simulink model "equivalent"  (R2018a)
settings: Solver=VariableStepAuto  StartTime=0.0  StopTime=10.0  RelTol=1e-3
undefined symbols (not defined in the file): DiscIntNeverNeededParam, sigbuilder_block
libraries: simulink x479
(part 3 of 10)

== system equivalent/cfblk303 ==
  cfblk1 : Inport
  cfblk9 : Inport  Port=2
  Action Port : ActionPort  ActionType=then
  cfblk10 : Subsystem  TreatAsAtomicUnit=on
  cfblk11 : Subsystem  TreatAsAtomicUnit=on
  cfblk12 : Delay
  cfblk13 : Delay
  cfblk3 : DiscreteZeroPole  Poles=[0 0.5]  Gain=1  SampleTime=-1
  cfblk4 : UnitDelay  SampleTime=-1
  cfblk5 : simulink/Discrete/Tapped Delay  vinit=0.0  samptime=-1  NumDelays=1  DelayOrder=Oldest  includeCurrent=off
  cfblk6 : simulink/Discrete/Transfer Fcn Lead or Lag  PoleZ=0.95  ZeroZ=0.75  ICPrevOutput=0.0  ICPrevInput=0.0  DoSatur=off
      settings: SourceProductName=Simulink  SourceProductBaseCode=SL
  cfblk7 : simulink/Discrete/Transfer Fcn Lead or Lag  PoleZ=0.95  ZeroZ=0.75  ICPrevOutput=0.0  ICPrevInput=0.0  DoSatur=off
      settings: SourceProductName=Simulink  SourceProductBaseCode=SL
  cfblk8 : If  SampleTime=1
  cyemi_{597..600,612..613,626..633} (14 alike) : DataTypeConversion  OutDataTypeStr=double
  cfblk2 : Outport
  wires:
  cfblk7/1 -> cyemi_613/1, cyemi_633/1
  cfblk1/1 -> cyemi_600/1, cyemi_630/1
  cfblk10/1(cfblk2) -> cfblk2/1
  cfblk8/1 -> cfblk10/Action
  cfblk8/2 -> cfblk11/Action
  cyemi_597/1 -> cfblk10/1(cfblk1)
  cfblk3/1 -> cyemi_597/1
  cyemi_598/1 -> cfblk10/2(cfblk12)
  cfblk12/1 -> cyemi_598/1
  cyemi_599/1 -> cfblk10/3(cfblk13)
  cfblk13/1 -> cyemi_599/1
  cyemi_600/1 -> cfblk10/4(cfblk14)
  cyemi_612/1 -> cfblk11/1(cfblk1)
  cfblk10/2(cfblk15) -> cyemi_612/1
  cyemi_613/1 -> cfblk11/2(cfblk13)
  cyemi_626/1 -> cfblk12/1
  cfblk11/1(cfblk2) -> cyemi_626/1
  cyemi_627/1 -> cfblk13/1
  cfblk11/2(cfblk14) -> cyemi_627/1
  cyemi_628/1 -> cfblk3/1
  cfblk5/1 -> cyemi_628/1
  cyemi_629/1 -> cfblk4/1
  cfblk6/1 -> cyemi_629/1
  cyemi_630/1 -> cfblk5/1
  cyemi_631/1 -> cfblk6/1
  cfblk9/1 -> cyemi_631/1
  cyemi_632/1 -> cfblk7/1
  cfblk4/1 -> cyemi_632/1
  cyemi_633/1 -> cfblk8/1

== system equivalent/cfblk304 ==
  cfblk1 : Inport
  cfblk7 : Inport  Port=2
  Action Port : ActionPort  ActionType=else
  cfblk10 : Subsystem  TreatAsAtomicUnit=on
  cfblk11 : Subsystem  TreatAsAtomicUnit=on
  cfblk12 : Delay
  cfblk13 : Delay
  cfblk3 : DiscreteTransferFcn
  cfblk4 : DiscreteFir
  cfblk5 : simulink/Continuous/PID Controller  Controller=PID  TimeDomain=Discrete-time  SampleTime=-1  IntegratorMethod=Forward Euler  FilterMethod=Forward Euler  Form=Parallel  UseFilter=on  ControllerParametersSource=internal  P=1  I=1  D=0  N=100  InitialConditionSource=internal  InitialConditionForIntegrator=0  InitialConditionForFilter=0  ExternalReset=none  LimitOutput=off  UpperSaturationLimit=inf  LowerSaturationLimit=-inf  LinearizeAsGain=off  AntiWindupMode=none  Kb=1  TrackingMode=off  Kt=1  PParamMin=[]  PParamMax=[]  IParamMin=[]  IParamMax=[]  DParamMin=[]  DParamMax=[]  NParamMin=[]  NParamMax=[]  KbParamMin=[]  KbParamMax=[]  KtParamMin=[]  KtParamMax=[]  POutMin=[]  POutMax=[]  IOutMin=[]  IOutMax=[]  DOutMin=[]  DOutMax=[]  NOutMin=[]  NOutMax=[]  KbOutMin=[]  KbOutMax=[]  KtOutMin=[]  KtOutMax=[]  IntegratorOutMin=[]  IntegratorOutMax=[]  FilterOutMin=[]  FilterOutMax=[]  SumOutMin=[]  SumOutMax=[]  SumI1OutMin=[]  SumI1OutMax=[]  SumI2OutMin=[]  SumI2OutMax=[]  SumI3OutMin=[]  SumI3OutMax=[]  SumDOutMin=[]  SumDOutMax=[]  SaturationOutMin=[]  SaturationOutMax=[]  IntegratorContinuousStateAttributes=''  IntegratorStateMustResolveToSignalObject=off  IntegratorRTWStateStorageClass=Auto  FilterContinuousStateAttributes=''  FilterStateMustResolveToSignalObject=off  FilterRTWStateStorageClass=Auto  DifferentiatorICPrevScaledInput=0  DifferentiatorOutMin=[]  DifferentiatorOutMax=[]  FilterDiffOutCoefMin=[]  FilterDiffOutCoefMax=[]  SumDenOutMin=[]  SumDenOutMax=[]  SumNumOutMin=[]  SumNumOutMax=[]  ReciprocalOutMin=[]  ReciprocalOutMax=[]  DivideOutMin=[]  DivideOutMax=[]  TunerSelectOption=Transfer Function Based (PID Tuner App)
  cfblk6 : If  SampleTime=1
  cyemi_{636..637,650,657..662} (9 alike) : DataTypeConversion  OutDataTypeStr=double
  cfblk2 : Outport
  cfblk8 : Outport  Port=2
  cfblk9 : Outport  Port=3
  wires:
  cfblk4/1 -> cfblk8/1, cyemi_637/1
  cfblk5/1 -> cfblk2/1
  cfblk11/1(cfblk2) -> cfblk9/1
  cfblk11/2(cfblk7) -> cyemi_636/1, cyemi_658/1
  cfblk6/1 -> cfblk10/Action
  cfblk6/2 -> cfblk11/Action
  cyemi_636/1 -> cfblk10/1(cfblk1)
  cyemi_637/1 -> cfblk10/2(cfblk12)
  cyemi_650/1 -> cfblk11/1(cfblk1)
  cfblk7/1 -> cyemi_650/1
  cyemi_657/1 -> cfblk12/1
  cfblk10/1(cfblk2) -> cyemi_657/1
  cyemi_658/1 -> cfblk13/1
  cyemi_659/1 -> cfblk3/1
  cfblk1/1 -> cyemi_659/1
  cyemi_660/1 -> cfblk4/1
  cfblk12/1 -> cyemi_660/1
  cyemi_661/1 -> cfblk5/1
  cfblk3/1 -> cyemi_661/1
  cyemi_662/1 -> cfblk6/1
  cfblk13/1 -> cyemi_662/1

== system equivalent/cfblk305 ==
  cfblk1 : Inport
  cfblk9 : Inport  Port=2
  cfblk10 : Inport  Port=3
  cfblk11 : Inport  Port=4
  cfblk12 : Inport  Port=5
  Action Port : ActionPort  ActionType=then
  cfblk14 : Subsystem  TreatAsAtomicUnit=on
  cfblk15 : Subsystem  TreatAsAtomicUnit=on
  cfblk16 : Delay
  cfblk3 : DiscreteFir
  cfblk4 : DiscreteStateSpace  SampleTime=-1
  cfblk5 : simulink/Discrete/Tapped Delay  vinit=0.0  samptime=-1  NumDelays=1  DelayOrder=Oldest  includeCurrent=off
  cfblk6 : simulink/Discrete/Transfer Fcn Lead or Lag  PoleZ=0.95  ZeroZ=0.75  ICPrevOutput=0.0  ICPrevInput=0.0  DoSatur=off
      settings: SourceProductName=Simulink  SourceProductBaseCode=SL
  cfblk7 : simulink/Discrete/Transfer Fcn First Order  PoleZ=0.95  ICPrevOutput=0.0  DoSatur=off
      settings: SourceProductName=Simulink
  cfblk8 : If  SampleTime=1
  cyemi_{668,678..681,698..704} (12 alike) : DataTypeConversion  OutDataTypeStr=double
  cfblk2 : Outport
  cfblk13 : Outport  Port=2
  wires:
  cfblk14/1(cfblk2) -> cfblk13/1
  cfblk15/1(cfblk2) -> cfblk2/1
  cfblk8/1 -> cfblk14/Action
  cfblk8/2 -> cfblk15/Action
  cyemi_668/1 -> cfblk14/1(cfblk1)
  cfblk7/1 -> cyemi_668/1
  cyemi_678/1 -> cfblk15/1(cfblk1)
  cfblk6/1 -> cyemi_678/1
  cyemi_679/1 -> cfblk15/2(cfblk14)
  cfblk4/1 -> cyemi_679/1
  cyemi_680/1 -> cfblk15/3(cfblk15)
  cfblk5/1 -> cyemi_680/1
  cyemi_681/1 -> cfblk15/4(cfblk16)
  cfblk9/1 -> cyemi_681/1
  cyemi_698/1 -> cfblk16/1
  cfblk15/2(cfblk17) -> cyemi_698/1
  cyemi_699/1 -> cfblk3/1
  cfblk16/1 -> cyemi_699/1
  cyemi_700/1 -> cfblk4/1
  cfblk12/1 -> cyemi_700/1
  cyemi_701/1 -> cfblk5/1
  cfblk10/1 -> cyemi_701/1
  cyemi_702/1 -> cfblk6/1
  cfblk3/1 -> cyemi_702/1
  cyemi_703/1 -> cfblk7/1
  cfblk1/1 -> cyemi_703/1
  cyemi_704/1 -> cfblk8/1
  cfblk11/1 -> cyemi_704/1

== system equivalent/cfblk306 ==
  cfblk1 : Inport
  Action Port : ActionPort  ActionType=else
  cfblk10 : DiscreteFir
  cfblk11 : DiscreteZeroPole  Poles=[0 0.5]  Gain=1  SampleTime=-1
  cfblk13 : Delay
  cfblk14 : Delay
  cfblk3 : Delay  ShowEnablePort=on
      settings: InputPortMap=u0,e6
  cfblk4 : DiscreteTransferFcn
  cfblk5 : Delay  ShowEnablePort=on
      settings: InputPortMap=u0,e6
  cfblk6 : Delay  DelayLengthSource=Input port
      settings: InputPortMap=u0,p1
  cfblk7 : Delay  DelayLengthSource=Input port
      settings: InputPortMap=u0,p1
  cfblk8 : Delay  DelayLengthSource=Input port
      settings: InputPortMap=u0,p1
  cfblk9 : simulink/Continuous/PID Controller (2DOF)  Controller=PID  TimeDomain=Discrete-time  SampleTime=-1  IntegratorMethod=Forward Euler  FilterMethod=Forward Euler  Form=Parallel  UseFilter=on  ControllerParametersSource=internal  P=1  I=1  D=0  N=100  b=1  c=1  InitialConditionSource=internal  InitialConditionForIntegrator=0  InitialConditionForFilter=0  ExternalReset=none  LimitOutput=off  UpperSaturationLimit=inf  LowerSaturationLimit=-inf  LinearizeAsGain=off  AntiWindupMode=none  Kb=1  TrackingMode=off  Kt=1  PParamMin=[]  PParamMax=[]  IParamMin=[]  IParamMax=[]  DParamMin=[]  DParamMax=[]  NParamMin=[]  NParamMax=[]  bParamMin=[]  bParamMax=[]  cParamMin=[]  cParamMax=[]  KbParamMin=[]  KbParamMax=[]  KtParamMin=[]  KtParamMax=[]  POutMin=[]  POutMax=[]  IOutMin=[]  IOutMax=[]  DOutMin=[]  DOutMax=[]  NOutMin=[]  NOutMax=[]  bOutMin=[]  bOutMax=[]  cOutMin=[]  cOutMax=[]  KbOutMin=[]  KbOutMax=[]  KtOutMin=[]  KtOutMax=[]  IntegratorOutMin=[]  IntegratorOutMax=[]  FilterOutMin=[]  FilterOutMax=[]  SumOutMin=[]  SumOutMax=[]  Sum1OutMin=[]  Sum1OutMax=[]  Sum2OutMin=[]  Sum2OutMax=[]  Sum3OutMin=[]  Sum3OutMax=[]  SumI1OutMin=[]  SumI1OutMax=[]  SumI2OutMin=[]  SumI2OutMax=[]  SumI3OutMin=[]  SumI3OutMax=[]  SumDOutMin=[]  SumDOutMax=[]  SaturationOutMin=[]  SaturationOutMax=[]  IntegratorContinuousStateAttributes=''  IntegratorStateMustResolveToSignalObject=off  IntegratorRTWStateStorageClass=Auto  FilterContinuousStateAttributes=''  FilterStateMustResolveToSignalObject=off  FilterRTWStateStorageClass=Auto  DifferentiatorICPrevScaledInput=0  DifferentiatorOutMin=[]  DifferentiatorOutMax=[]  FilterDiffOutCoefMin=[]  FilterDiffOutCoefMax=[]  SumDenOutMin=[]  SumDenOutMax=[]  SumNumOutMin=[]  SumNumOutMax=[]  ReciprocalOutMin=[]  ReciprocalOutMax=[]  DivideOutMin=[]  DivideOutMax=[]  TunerSelectOption=Transfer Function Based (PID Tuner App)
  cyemi_{706..722} (17 alike) : DataTypeConversion  OutDataTypeStr=double
  cfblk2 : Outport
  cfblk12 : Outport  Port=2
  wires:
  cfblk9/1 -> cfblk2/1, cyemi_718/1
  cfblk5/1 -> cyemi_710/1, cyemi_712/1
  cfblk3/1 -> cfblk12/1, cyemi_716/1
  cfblk4/1 -> cyemi_707/1, cyemi_719/1
  cfblk1/1 -> cyemi_713/1, cyemi_720/1
  cfblk10/1 -> cyemi_709/1, cyemi_711/1, cyemi_721/1
  cyemi_706/1 -> cfblk10/1
  cfblk11/1 -> cyemi_706/1
  cyemi_707/1 -> cfblk11/1
  cyemi_708/1 -> cfblk13/1
  cfblk7/1 -> cyemi_708/1
  cyemi_709/1 -> cfblk14/1
  cyemi_710/1 -> cfblk3/1
  cyemi_711/1 -> cfblk3/2
  cyemi_712/1 -> cfblk4/1
  cyemi_713/1 -> cfblk5/1
  cyemi_714/1 -> cfblk5/2
  cfblk14/1 -> cyemi_714/1
  cyemi_715/1 -> cfblk6/1
  cfblk13/1 -> cyemi_715/1
  cyemi_716/1 -> cfblk6/2
  cyemi_717/1 -> cfblk7/1
  cfblk6/1 -> cyemi_717/1
  cyemi_718/1 -> cfblk7/2
  cyemi_719/1 -> cfblk8/1
  cyemi_720/1 -> cfblk8/2
  cyemi_721/1 -> cfblk9/1
  cyemi_722/1 -> cfblk9/2
  cfblk8/1 -> cyemi_722/1

== system equivalent/cfblk307 ==
  cfblk1 : Inport
  cfblk12 : Inport  Port=2
  cfblk13 : Inport  Port=3
  cfblk14 : Inport  Port=4
  cfblk15 : Inport  Port=5
  cfblk16 : Inport  Port=6
  Action Port : ActionPort  ActionType=then
  cfblk10 : simulink/Discrete/Transfer Fcn Real Zero  ZeroZ=0.75  ICPrevInput=0.0  DoSatur=off
      settings: SourceProductName=Simulink  SourceProductBaseCode=SL
  cfblk11 : simulink/Discrete/Transfer Fcn Real Zero  ZeroZ=0.75  ICPrevInput=0.0  DoSatur=off
      settings: SourceProductName=Simulink  SourceProductBaseCode=SL
  cfblk{7..9,17} (4 alike) : Delay
  cfblk3 : DiscreteFilter
  cfblk4 : DiscreteFir
  cfblk5 : DiscreteIntegrator  SampleTime=-1  ICPrevOutput=DiscIntNeverNeededParam  ICPrevScaledInput=DiscIntNeverNeededParam
  cfblk6 : simulink/Discrete/Transfer Fcn First Order  PoleZ=0.95  ICPrevOutput=0.0  DoSatur=off
      settings: SourceProductName=Simulink
  cyemi_{729..738} (10 alike) : DataTypeConversion  OutDataTypeStr=double
  cfblk2 : Outport
  wires:
  cfblk15/1 -> cfblk2/1
  cyemi_729/1 -> cfblk10/1
  cfblk7/1 -> cyemi_729/1
  cyemi_730/1 -> cfblk11/1
  cfblk14/1 -> cyemi_730/1
  cyemi_731/1 -> cfblk17/1
  cfblk6/1 -> cyemi_731/1
  cyemi_732/1 -> cfblk3/1
  cfblk1/1 -> cyemi_732/1
  cyemi_733/1 -> cfblk4/1
  cfblk17/1 -> cyemi_733/1
  cyemi_734/1 -> cfblk5/1
  cfblk12/1 -> cyemi_734/1
  cyemi_735/1 -> cfblk6/1
  cfblk4/1 -> cyemi_735/1
  cyemi_736/1 -> cfblk7/1
  cfblk16/1 -> cyemi_736/1
  cyemi_737/1 -> cfblk8/1
  cfblk11/1 -> cyemi_737/1
  cyemi_738/1 -> cfblk9/1
  cfblk8/1 -> cyemi_738/1

== system equivalent/cfblk308 ==
  cfblk1 : Inport
  cfblk10 : Inport  Port=2
  Action Port : ActionPort  ActionType=else
  cfblk11 : Subsystem  TreatAsAtomicUnit=on
  cfblk12 : Subsystem  TreatAsAtomicUnit=on
  cfblk{13..16} (4 alike) : Delay
  cfblk3 : DiscreteIntegrator  SampleTime=-1  ICPrevOutput=DiscIntNeverNeededParam  ICPrevScaledInput=DiscIntNeverNeededParam
  cfblk4 : simulink/Continuous/PID Controller (2DOF)  Controller=PID  TimeDomain=Discrete-time  SampleTime=-1  IntegratorMethod=Forward Euler  FilterMethod=Forward Euler  Form=Parallel  UseFilter=on  ControllerParametersSource=internal  P=1  I=1  D=0  N=100  b=1  c=1  InitialConditionSource=internal  InitialConditionForIntegrator=0  InitialConditionForFilter=0  ExternalReset=none  LimitOutput=off  UpperSaturationLimit=inf  LowerSaturationLimit=-inf  LinearizeAsGain=off  AntiWindupMode=none  Kb=1  TrackingMode=off  Kt=1  PParamMin=[]  PParamMax=[]  IParamMin=[]  IParamMax=[]  DParamMin=[]  DParamMax=[]  NParamMin=[]  NParamMax=[]  bParamMin=[]  bParamMax=[]  cParamMin=[]  cParamMax=[]  KbParamMin=[]  KbParamMax=[]  KtParamMin=[]  KtParamMax=[]  POutMin=[]  POutMax=[]  IOutMin=[]  IOutMax=[]  DOutMin=[]  DOutMax=[]  NOutMin=[]  NOutMax=[]  bOutMin=[]  bOutMax=[]  cOutMin=[]  cOutMax=[]  KbOutMin=[]  KbOutMax=[]  KtOutMin=[]  KtOutMax=[]  IntegratorOutMin=[]  IntegratorOutMax=[]  FilterOutMin=[]  FilterOutMax=[]  SumOutMin=[]  SumOutMax=[]  Sum1OutMin=[]  Sum1OutMax=[]  Sum2OutMin=[]  Sum2OutMax=[]  Sum3OutMin=[]  Sum3OutMax=[]  SumI1OutMin=[]  SumI1OutMax=[]  SumI2OutMin=[]  SumI2OutMax=[]  SumI3OutMin=[]  SumI3OutMax=[]  SumDOutMin=[]  SumDOutMax=[]  SaturationOutMin=[]  SaturationOutMax=[]  IntegratorContinuousStateAttributes=''  IntegratorStateMustResolveToSignalObject=off  IntegratorRTWStateStorageClass=Auto  FilterContinuousStateAttributes=''  FilterStateMustResolveToSignalObject=off  FilterRTWStateStorageClass=Auto  DifferentiatorICPrevScaledInput=0  DifferentiatorOutMin=[]  DifferentiatorOutMax=[]  FilterDiffOutCoefMin=[]  FilterDiffOutCoefMax=[]  SumDenOutMin=[]  SumDenOutMax=[]  SumNumOutMin=[]  SumNumOutMax=[]  ReciprocalOutMin=[]  ReciprocalOutMax=[]  DivideOutMin=[]  DivideOutMax=[]  TunerSelectOption=Transfer Function Based (PID Tuner App)
  cfblk5 : DiscreteZeroPole  Poles=[0 0.5]  Gain=1  SampleTime=-1
  cfblk6 : DiscreteFilter
  cfblk7 : DiscreteStateSpace  SampleTime=-1
  cfblk8 : simulink/Continuous/PID Controller  Controller=PID  TimeDomain=Discrete-time  SampleTime=-1  IntegratorMethod=Forward Euler  FilterMethod=Forward Euler  Form=Parallel  UseFilter=on  ControllerParametersSource=internal  P=1  I=1  D=0  N=100  InitialConditionSource=internal  InitialConditionForIntegrator=0  InitialConditionForFilter=0  ExternalReset=none  LimitOutput=off  UpperSaturationLimit=inf  LowerSaturationLimit=-inf  LinearizeAsGain=off  AntiWindupMode=none  Kb=1  TrackingMode=off  Kt=1  PParamMin=[]  PParamMax=[]  IParamMin=[]  IParamMax=[]  DParamMin=[]  DParamMax=[]  NParamMin=[]  NParamMax=[]  KbParamMin=[]  KbParamMax=[]  KtParamMin=[]  KtParamMax=[]  POutMin=[]  POutMax=[]  IOutMin=[]  IOutMax=[]  DOutMin=[]  DOutMax=[]  NOutMin=[]  NOutMax=[]  KbOutMin=[]  KbOutMax=[]  KtOutMin=[]  KtOutMax=[]  IntegratorOutMin=[]  IntegratorOutMax=[]  FilterOutMin=[]  FilterOutMax=[]  SumOutMin=[]  SumOutMax=[]  SumI1OutMin=[]  SumI1OutMax=[]  SumI2OutMin=[]  SumI2OutMax=[]  SumI3OutMin=[]  SumI3OutMax=[]  SumDOutMin=[]  SumDOutMax=[]  SaturationOutMin=[]  SaturationOutMax=[]  IntegratorContinuousStateAttributes=''  IntegratorStateMustResolveToSignalObject=off  IntegratorRTWStateStorageClass=Auto  FilterContinuousStateAttributes=''  FilterStateMustResolveToSignalObject=off  FilterRTWStateStorageClass=Auto  DifferentiatorICPrevScaledInput=0  DifferentiatorOutMin=[]  DifferentiatorOutMax=[]  FilterDiffOutCoefMin=[]  FilterDiffOutCoefMax=[]  SumDenOutMin=[]  SumDenOutMax=[]  SumNumOutMin=[]  SumNumOutMax=[]  ReciprocalOutMin=[]  ReciprocalOutMax=[]  DivideOutMin=[]  DivideOutMax=[]  TunerSelectOption=Transfer Function Based (PID Tuner App)
  cfblk9 : If  SampleTime=1
  cyemi_{741..742,750,761..772} (15 alike) : DataTypeConversion  OutDataTypeStr=double
  cfblk2 : Outport
  wires:
  cfblk1/1 -> cfblk2/1
  cfblk9/1 -> cfblk11/Action
  cfblk9/2 -> cfblk12/Action
  cyemi_741/1 -> cfblk11/1(cfblk1)
  cfblk13/1 -> cyemi_741/1
  cyemi_742/1 -> cfblk11/2(cfblk7)
  cfblk12/2(cfblk10) -> cyemi_742/1
  cyemi_750/1 -> cfblk12/1(cfblk1)
  cfblk3/1 -> cyemi_750/1
  cyemi_761/1 -> cfblk13/1
  cfblk4/1 -> cyemi_761/1
  cyemi_762/1 -> cfblk14/1
  cfblk11/1(cfblk2) -> cyemi_762/1
  cyemi_763/1 -> cfblk15/1
  cfblk7/1 -> cyemi_763/1
  cyemi_764/1 -> cfblk16/1
  cfblk6/1 -> cyemi_764/1
  cyemi_765/1 -> cfblk3/1
  cfblk8/1 -> cyemi_765/1
  cyemi_766/1 -> cfblk4/1
  cfblk12/1(cfblk2) -> cyemi_766/1
  cyemi_767/1 -> cfblk4/2
  cfblk14/1 -> cyemi_767/1
  cyemi_768/1 -> cfblk5/1
  cfblk16/1 -> cyemi_768/1
  cyemi_769/1 -> cfblk6/1
  cfblk5/1 -> cyemi_769/1
  cyemi_770/1 -> cfblk7/1
  cfblk12/3(cfblk11) -> cyemi_770/1
  cyemi_771/1 -> cfblk8/1
  cfblk10/1 -> cyemi_771/1
  cyemi_772/1 -> cfblk9/1
  cfblk15/1 -> cyemi_772/1

== system equivalent/cfblk309 ==
  cfblk1 : Inport
  cfblk13 : Inport  Port=2
  Action Port : ActionPort  ActionType=then
  cfblk10 : simulink/Continuous/PID Controller (2DOF)  Controller=PID  TimeDomain=Discrete-time  SampleTime=-1  IntegratorMethod=Forward Euler  FilterMethod=Forward Euler  Form=Parallel  UseFilter=on  ControllerParametersSource=internal  P=1  I=1  D=0  N=100  b=1  c=1  InitialConditionSource=internal  InitialConditionForIntegrator=0  InitialConditionForFilter=0  ExternalReset=none  LimitOutput=off  UpperSaturationLimit=inf  LowerSaturationLimit=-inf  LinearizeAsGain=off  AntiWindupMode=none  Kb=1  TrackingMode=off  Kt=1  PParamMin=[]  PParamMax=[]  IParamMin=[]  IParamMax=[]  DParamMin=[]  DParamMax=[]  NParamMin=[]  NParamMax=[]  bParamMin=[]  bParamMax=[]  cParamMin=[]  cParamMax=[]  KbParamMin=[]  KbParamMax=[]  KtParamMin=[]  KtParamMax=[]  POutMin=[]  POutMax=[]  IOutMin=[]  IOutMax=[]  DOutMin=[]  DOutMax=[]  NOutMin=[]  NOutMax=[]  bOutMin=[]  bOutMax=[]  cOutMin=[]  cOutMax=[]  KbOutMin=[]  KbOutMax=[]  KtOutMin=[]  KtOutMax=[]  IntegratorOutMin=[]  IntegratorOutMax=[]  FilterOutMin=[]  FilterOutMax=[]  SumOutMin=[]  SumOutMax=[]  Sum1OutMin=[]  Sum1OutMax=[]  Sum2OutMin=[]  Sum2OutMax=[]  Sum3OutMin=[]  Sum3OutMax=[]  SumI1OutMin=[]  SumI1OutMax=[]  SumI2OutMin=[]  SumI2OutMax=[]  SumI3OutMin=[]  SumI3OutMax=[]  SumDOutMin=[]  SumDOutMax=[]  SaturationOutMin=[]  SaturationOutMax=[]  IntegratorContinuousStateAttributes=''  IntegratorStateMustResolveToSignalObject=off  IntegratorRTWStateStorageClass=Auto  FilterContinuousStateAttributes=''  FilterStateMustResolveToSignalObject=off  FilterRTWStateStorageClass=Auto  DifferentiatorICPrevScaledInput=0  DifferentiatorOutMin=[]  DifferentiatorOutMax=[]  FilterDiffOutCoefMin=[]  FilterDiffOutCoefMax=[]  SumDenOutMin=[]  SumDenOutMax=[]  SumNumOutMin=[]  SumNumOutMax=[]  ReciprocalOutMin=[]  ReciprocalOutMax=[]  DivideOutMin=[]  DivideOutMax=[]  TunerSelectOption=Transfer Function Based (PID Tuner App)
  cfblk11 : DiscreteFilter
  cfblk12 : Delay
  cfblk15 : Delay
  cfblk3 : Delay  DelayLengthSource=Input port
      settings: InputPortMap=u0,p1
  cfblk4 : UnitDelay  SampleTime=-1
  cfblk5 : DiscreteStateSpace  SampleTime=-1
  cfblk6 : DiscreteZeroPole  Poles=[0 0.5]  Gain=1  SampleTime=-1
  cfblk7 : Delay  ShowEnablePort=on
      settings: InputPortMap=u0,e6
  cfblk8 : simulink/Discrete/Difference  ICPrevInput=0.0  OutMin=[]  OutMax=[]  OutDataTypeStr=Inherit: Inherit via back propagation  OutDataType=fixdt(1, 16)  OutScaling=2^-10  DoSatur=off
  cfblk9 : DiscreteTransferFcn
  cyemi_{775..788} (14 alike) : DataTypeConversion  OutDataTypeStr=double
  cfblk2 : Outport
  cfblk14 : Outport  Port=2
  wires:
  cfblk9/1 -> cyemi_785/1, cyemi_787/1
  cfblk3/1 -> cyemi_777/1, cyemi_778/1
  cfblk4/1 -> cfblk14/1
  cfblk5/1 -> cfblk2/1
  cfblk11/1 -> cyemi_786/1, cyemi_788/1
  cyemi_775/1 -> cfblk10/1
  cfblk13/1 -> cyemi_775/1
  cyemi_776/1 -> cfblk10/2
  cfblk6/1 -> cyemi_776/1
  cyemi_777/1 -> cfblk11/1
  cyemi_778/1 -> cfblk12/1
  cyemi_779/1 -> cfblk15/1
  cfblk10/1 -> cyemi_779/1
  cyemi_780/1 -> cfblk3/1
  cfblk15/1 -> cyemi_780/1
  cyemi_781/1 -> cfblk3/2
  cfblk1/1 -> cyemi_781/1
  cyemi_782/1 -> cfblk4/1
  cfblk7/1 -> cyemi_782/1
  cyemi_783/1 -> cfblk5/1
  cfblk8/1 -> cyemi_783/1
  cyemi_784/1 -> cfblk6/1
  cfblk12/1 -> cyemi_784/1
  cyemi_785/1 -> cfblk7/1
  cyemi_786/1 -> cfblk7/2
  cyemi_787/1 -> cfblk8/1
  cyemi_788/1 -> cfblk9/1

== system equivalent/cfblk310 ==
  cfblk1 : Inport
  cfblk13 : Inport  Port=2
  Action Port : ActionPort  ActionType=else
  cfblk10 : UnitDelay  SampleTime=-1
  cfblk11 : UnitDelay  SampleTime=-1
  cfblk12 : simulink/Discrete/Tapped Delay  vinit=0.0  samptime=-1  NumDelays=1  DelayOrder=Oldest  includeCurrent=off
  cfblk17 : Delay
  cfblk18 : Delay
  cfblk3 : Delay  DelayLengthSource=Input port
      settings: InputPortMap=u0,p1
  cfblk4 : DiscreteFilter
  cfblk5 : Delay
  cfblk6 : DiscreteTransferFcn
  cfblk7 : DiscreteStateSpace  SampleTime=-1
  cfblk8 : simulink/Discrete/Tapped Delay  vinit=0.0  samptime=-1  NumDelays=1  DelayOrder=Oldest  includeCurrent=off
  cfblk9 : simulink/Discrete/Tapped Delay  vinit=0.0  samptime=-1  NumDelays=1  DelayOrder=Oldest  includeCurrent=off
  cyemi_{792..804} (13 alike) : DataTypeConversion  OutDataTypeStr=double
  cfblk2 : Outport
  cfblk14 : Outport  Port=2
  cfblk15 : Outport  Port=3
  cfblk16 : Outport  Port=4
  wires:
  cfblk8/1 -> cfblk15/1
  cfblk5/1 -> cyemi_803/1, cyemi_804/1
  cfblk11/1 -> cyemi_795/1, cyemi_796/1, cyemi_802/1
  cfblk1/1 -> cfblk2/1
  cfblk7/1 -> cfblk16/1
  cfblk12/1 -> cfblk14/1
  cyemi_792/1 -> cfblk10/1
  cfblk3/1 -> cyemi_792/1
  cyemi_793/1 -> cfblk11/1
  cfblk10/1 -> cyemi_793/1
  cyemi_794/1 -> cfblk12/1
  cfblk4/1 -> cyemi_794/1
  cyemi_795/1 -> cfblk17/1
  cyemi_796/1 -> cfblk18/1
  cyemi_797/1 -> cfblk3/1
  cfblk17/1 -> cyemi_797/1
  cyemi_798/1 -> cfblk3/2
  cfblk18/1 -> cyemi_798/1
  cyemi_799/1 -> cfblk4/1
  cfblk9/1 -> cyemi_799/1
  cyemi_800/1 -> cfblk5/1
  cfblk6/1 -> cyemi_800/1
  cyemi_801/1 -> cfblk6/1
  cfblk13/1 -> cyemi_801/1
  cyemi_802/1 -> cfblk7/1
  cyemi_803/1 -> cfblk8/1
  cyemi_804/1 -> cfblk9/1

== system equivalent/cfblk311 ==
  cfblk1 : Inport
  cfblk9 : Inport  Port=2
  cfblk10 : Inport  Port=3
  cfblk11 : Inport  Port=4
  Action Port : ActionPort  ActionType=then
  cfblk3 : DiscreteFilter
  cfblk4 : DiscreteFir
  cfblk5 : simulink/Continuous/PID Controller (2DOF)  Controller=PID  TimeDomain=Discrete-time  SampleTime=-1  IntegratorMethod=Forward Euler  FilterMethod=Forward Euler  Form=Parallel  UseFilter=on  ControllerParametersSource=internal  P=1  I=1  D=0  N=100  b=1  c=1  InitialConditionSource=internal  InitialConditionForIntegrator=0  InitialConditionForFilter=0  ExternalReset=none  LimitOutput=off  UpperSaturationLimit=inf  LowerSaturationLimit=-inf  LinearizeAsGain=off  AntiWindupMode=none  Kb=1  TrackingMode=off  Kt=1  PParamMin=[]  PParamMax=[]  IParamMin=[]  IParamMax=[]  DParamMin=[]  DParamMax=[]  NParamMin=[]  NParamMax=[]  bParamMin=[]  bParamMax=[]  cParamMin=[]  cParamMax=[]  KbParamMin=[]  KbParamMax=[]  KtParamMin=[]  KtParamMax=[]  POutMin=[]  POutMax=[]  IOutMin=[]  IOutMax=[]  DOutMin=[]  DOutMax=[]  NOutMin=[]  NOutMax=[]  bOutMin=[]  bOutMax=[]  cOutMin=[]  cOutMax=[]  KbOutMin=[]  KbOutMax=[]  KtOutMin=[]  KtOutMax=[]  IntegratorOutMin=[]  IntegratorOutMax=[]  FilterOutMin=[]  FilterOutMax=[]  SumOutMin=[]  SumOutMax=[]  Sum1OutMin=[]  Sum1OutMax=[]  Sum2OutMin=[]  Sum2OutMax=[]  Sum3OutMin=[]  Sum3OutMax=[]  SumI1OutMin=[]  SumI1OutMax=[]  SumI2OutMin=[]  SumI2OutMax=[]  SumI3OutMin=[]  SumI3OutMax=[]  SumDOutMin=[]  SumDOutMax=[]  SaturationOutMin=[]  SaturationOutMax=[]  IntegratorContinuousStateAttributes=''  IntegratorStateMustResolveToSignalObject=off  IntegratorRTWStateStorageClass=Auto  FilterContinuousStateAttributes=''  FilterStateMustResolveToSignalObject=off  FilterRTWStateStorageClass=Auto  DifferentiatorICPrevScaledInput=0  DifferentiatorOutMin=[]  DifferentiatorOutMax=[]  FilterDiffOutCoefMin=[]  FilterDiffOutCoefMax=[]  SumDenOutMin=[]  SumDenOutMax=[]  SumNumOutMin=[]  SumNumOutMax=[]  ReciprocalOutMin=[]  ReciprocalOutMax=[]  DivideOutMin=[]  DivideOutMax=[]  TunerSelectOption=Transfer Function Based (PID Tuner App)
  cfblk6 : simulink/Discrete/Transfer Fcn Lead or Lag  PoleZ=0.95  ZeroZ=0.75  ICPrevOutput=0.0  ICPrevInput=0.0  DoSatur=off
      settings: SourceProductName=Simulink  SourceProductBaseCode=SL
  cfblk7 : UnitDelay  SampleTime=-1
  cfblk8 : DiscreteIntegrator  SampleTime=-1  ICPrevOutput=DiscIntNeverNeededParam  ICPrevScaledInput=DiscIntNeverNeededParam
  cyemi_{809..815} (7 alike) : DataTypeConversion  OutDataTypeStr=double
  cfblk2 : Outport
  cfblk12 : Outport  Port=2
  cfblk13 : Outport  Port=3
  wires:
  cfblk11/1 -> cfblk12/1
  cfblk4/1 -> cfblk2/1
  cfblk3/1 -> cfblk13/1
  cyemi_809/1 -> cfblk3/1
  cfblk1/1 -> cyemi_809/1
  cyemi_810/1 -> cfblk4/1
  cfblk6/1 -> cyemi_810/1
  cyemi_811/1 -> cfblk5/1
  cfblk9/1 -> cyemi_811/1
  cyemi_812/1 -> cfblk5/2
  cfblk7/1 -> cyemi_812/1
  cyemi_813/1 -> cfblk6/1
  cfblk5/1 -> cyemi_813/1
  cyemi_814/1 -> cfblk7/1
  cfblk8/1 -> cyemi_814/1
  cyemi_815/1 -> cfblk8/1
  cfblk10/1 -> cyemi_815/1

== system equivalent/cfblk312 ==
  cfblk1 : Inport
  cfblk10 : Inport  Port=2
  Action Port : ActionPort  ActionType=else
  cfblk11 : Delay
  cfblk3 : Delay  ShowEnablePort=on
      settings: InputPortMap=u0,e6
  cfblk4 : simulink/Discrete/Transfer Fcn Lead or Lag  PoleZ=0.95  ZeroZ=0.75  ICPrevOutput=0.0  ICPrevInput=0.0  DoSatur=off
      settings: SourceProductName=Simulink  SourceProductBaseCode=SL
  cfblk5 : UnitDelay  SampleTime=-1
  cfblk6 : simulink/Discrete/Transfer Fcn Real Zero  ZeroZ=0.75  ICPrevInput=0.0  DoSatur=off
      settings: SourceProductName=Simulink  SourceProductBaseCode=SL
  cfblk7 : DiscreteStateSpace  SampleTime=-1
  cfblk8 : simulink/Discrete/Transfer Fcn Lead or Lag  PoleZ=0.95  ZeroZ=0.75  ICPrevOutput=0.0  ICPrevInput=0.0  DoSatur=off
      settings: SourceProductName=Simulink  SourceProductBaseCode=SL
  cfblk9 : UnitDelay  SampleTime=-1
  cyemi_{818..826} (9 alike) : DataTypeConversion  OutDataTypeStr=double
  cfblk2 : Outport
  wires:
  cfblk4/1 -> cfblk2/1
  cyemi_818/1 -> cfblk11/1
  cfblk7/1 -> cyemi_818/1
  cyemi_819/1 -> cfblk3/1
  cfblk10/1 -> cyemi_819/1
  cyemi_820/1 -> cfblk3/2
  cfblk11/1 -> cyemi_820/1
  cyemi_821/1 -> cfblk4/1
  cfblk8/1 -> cyemi_821/1
  cyemi_822/1 -> cfblk5/1
  cfblk3/1 -> cyemi_822/1
  cyemi_823/1 -> cfblk6/1
  cfblk5/1 -> cyemi_823/1
  cyemi_824/1 -> cfblk7/1
  cfblk6/1 -> cyemi_824/1
  cyemi_825/1 -> cfblk8/1
  cfblk9/1 -> cyemi_825/1
  cyemi_826/1 -> cfblk9/1
  cfblk1/1 -> cyemi_826/1

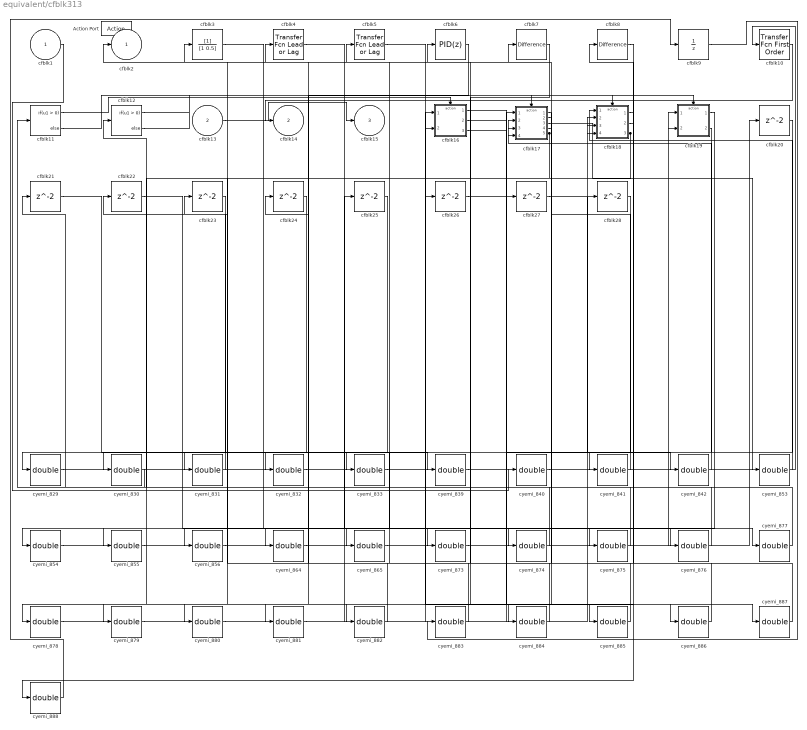
== system equivalent/cfblk313 ==
  cfblk1 : Inport
  cfblk13 : Inport  Port=2
  Action Port : ActionPort  ActionType=then
  cfblk10 : simulink/Discrete/Transfer Fcn First Order  PoleZ=0.95  ICPrevOutput=0.0  DoSatur=off
      settings: SourceProductName=Simulink
  cfblk11 : If  SampleTime=1
  cfblk12 : If  SampleTime=1
  cfblk16 : Subsystem  TreatAsAtomicUnit=on
  cfblk17 : Subsystem  TreatAsAtomicUnit=on
  cfblk18 : Subsystem  TreatAsAtomicUnit=on
  cfblk19 : Subsystem  TreatAsAtomicUnit=on
  cfblk{20..28} (9 alike) : Delay
  cfblk3 : DiscreteFilter
  cfblk4 : simulink/Discrete/Transfer Fcn Lead or Lag  PoleZ=0.95  ZeroZ=0.75  ICPrevOutput=0.0  ICPrevInput=0.0  DoSatur=off
      settings: SourceProductName=Simulink  SourceProductBaseCode=SL
  cfblk5 : simulink/Discrete/Transfer Fcn Lead or Lag  PoleZ=0.95  ZeroZ=0.75  ICPrevOutput=0.0  ICPrevInput=0.0  DoSatur=off
      settings: SourceProductName=Simulink  SourceProductBaseCode=SL
  cfblk6 : simulink/Continuous/PID Controller  Controller=PID  TimeDomain=Discrete-time  SampleTime=-1  IntegratorMethod=Forward Euler  FilterMethod=Forward Euler  Form=Parallel  UseFilter=on  ControllerParametersSource=internal  P=1  I=1  D=0  N=100  InitialConditionSource=internal  InitialConditionForIntegrator=0  InitialConditionForFilter=0  ExternalReset=none  LimitOutput=off  UpperSaturationLimit=inf  LowerSaturationLimit=-inf  LinearizeAsGain=off  AntiWindupMode=none  Kb=1  TrackingMode=off  Kt=1  PParamMin=[]  PParamMax=[]  IParamMin=[]  IParamMax=[]  DParamMin=[]  DParamMax=[]  NParamMin=[]  NParamMax=[]  KbParamMin=[]  KbParamMax=[]  KtParamMin=[]  KtParamMax=[]  POutMin=[]  POutMax=[]  IOutMin=[]  IOutMax=[]  DOutMin=[]  DOutMax=[]  NOutMin=[]  NOutMax=[]  KbOutMin=[]  KbOutMax=[]  KtOutMin=[]  KtOutMax=[]  IntegratorOutMin=[]  IntegratorOutMax=[]  FilterOutMin=[]  FilterOutMax=[]  SumOutMin=[]  SumOutMax=[]  SumI1OutMin=[]  SumI1OutMax=[]  SumI2OutMin=[]  SumI2OutMax=[]  SumI3OutMin=[]  SumI3OutMax=[]  SumDOutMin=[]  SumDOutMax=[]  SaturationOutMin=[]  SaturationOutMax=[]  IntegratorContinuousStateAttributes=''  IntegratorStateMustResolveToSignalObject=off  IntegratorRTWStateStorageClass=Auto  FilterContinuousStateAttributes=''  FilterStateMustResolveToSignalObject=off  FilterRTWStateStorageClass=Auto  DifferentiatorICPrevScaledInput=0  DifferentiatorOutMin=[]  DifferentiatorOutMax=[]  FilterDiffOutCoefMin=[]  FilterDiffOutCoefMax=[]  SumDenOutMin=[]  SumDenOutMax=[]  SumNumOutMin=[]  SumNumOutMax=[]  ReciprocalOutMin=[]  ReciprocalOutMax=[]  DivideOutMin=[]  DivideOutMax=[]  TunerSelectOption=Transfer Function Based (PID Tuner App)
  cfblk7 : simulink/Discrete/Difference  ICPrevInput=0.0  OutMin=[]  OutMax=[]  OutDataTypeStr=Inherit: Inherit via back propagation  OutDataType=fixdt(1, 16)  OutScaling=2^-10  DoSatur=off
  cfblk8 : simulink/Discrete/Difference  ICPrevInput=0.0  OutMin=[]  OutMax=[]  OutDataTypeStr=Inherit: Inherit via back propagation  OutDataType=fixdt(1, 16)  OutScaling=2^-10  DoSatur=off
  cfblk9 : UnitDelay  SampleTime=-1
  cyemi_{829..833,839..842,853..856,864..865,873..888} (31 alike) : DataTypeConversion  OutDataTypeStr=double
  cfblk2 : Outport
  cfblk14 : Outport  Port=2
  cfblk15 : Outport  Port=3
  wires:
  cfblk13/1 -> cfblk15/1
  cfblk17/2(cfblk13) -> cfblk2/1
  cfblk10/1 -> cfblk14/1
  cfblk17/5(cfblk16) -> cyemi_832/1, cyemi_856/1
  cfblk18/3(cfblk12) -> cyemi_879/1, cyemi_880/1
  cfblk11/1 -> cfblk16/Action
  cfblk11/2 -> cfblk17/Action
  cfblk12/1 -> cfblk18/Action
  cfblk12/2 -> cfblk19/Action
  cyemi_829/1 -> cfblk10/1
  cfblk19/2(cfblk10) -> cyemi_829/1
  cyemi_830/1 -> cfblk11/1
  cfblk24/1 -> cyemi_830/1
  cyemi_831/1 -> cfblk12/1
  cfblk17/1(cfblk2) -> cyemi_831/1
  cyemi_832/1 -> cfblk16/1(cfblk1)
  cyemi_833/1 -> cfblk16/2(cfblk7)
  cfblk25/1 -> cyemi_833/1
  cyemi_839/1 -> cfblk17/1(cfblk1)
  cfblk21/1 -> cyemi_839/1
  cyemi_840/1 -> cfblk17/2(cfblk10)
  cfblk1/1 -> cyemi_840/1
  cyemi_841/1 -> cfblk17/3(cfblk11)
  cfblk26/1 -> cyemi_841/1
  cyemi_842/1 -> cfblk17/4(cfblk12)
  cfblk27/1 -> cyemi_842/1
  cyemi_853/1 -> cfblk18/1(cfblk1)
  cfblk17/3(cfblk14) -> cyemi_853/1
  cyemi_854/1 -> cfblk18/2(cfblk8)
  cfblk17/4(cfblk15) -> cyemi_854/1
  cyemi_855/1 -> cfblk18/3(cfblk9)
  cfblk23/1 -> cyemi_855/1
  cyemi_856/1 -> cfblk18/4(cfblk10)
  cyemi_864/1 -> cfblk19/1(cfblk1)
  cfblk22/1 -> cyemi_864/1
  cyemi_865/1 -> cfblk19/2(cfblk9)
  cfblk20/1 -> cyemi_865/1
  cyemi_873/1 -> cfblk20/1
  cfblk3/1 -> cyemi_873/1
  cyemi_874/1 -> cfblk21/1
  cfblk19/1(cfblk2) -> cyemi_874/1
  cyemi_875/1 -> cfblk22/1
  cfblk16/2(cfblk8) -> cyemi_875/1
  cyemi_876/1 -> cfblk23/1
  cfblk16/3(cfblk9) -> cyemi_876/1
  cyemi_877/1 -> cfblk24/1
  cfblk4/1 -> cyemi_877/1
  cyemi_878/1 -> cfblk25/1
  cfblk18/2(cfblk11) -> cyemi_878/1
  cyemi_879/1 -> cfblk26/1
  cyemi_880/1 -> cfblk27/1
  cyemi_881/1 -> cfblk28/1
  cfblk6/1 -> cyemi_881/1
  cyemi_882/1 -> cfblk3/1
  cfblk7/1 -> cyemi_882/1
  cyemi_883/1 -> cfblk4/1
  cfblk9/1 -> cyemi_883/1
  cyemi_884/1 -> cfblk5/1
  cfblk28/1 -> cyemi_884/1
  cyemi_885/1 -> cfblk6/1
  cfblk8/1 -> cyemi_885/1
  cyemi_886/1 -> cfblk7/1
  cfblk16/1(cfblk2) -> cyemi_886/1
  cyemi_887/1 -> cfblk8/1
  cfblk5/1 -> cyemi_887/1
  cyemi_888/1 -> cfblk9/1
  cfblk18/1(cfblk2) -> cyemi_888/1

== system equivalent/cfblk314 ==
  cfblk1 : Inport
  Action Port : ActionPort  ActionType=else
  cfblk10 : Subsystem  TreatAsAtomicUnit=on
  cfblk11 : Subsystem  TreatAsAtomicUnit=on
  cfblk{12..15} (4 alike) : Delay
  cfblk3 : Delay  DelayLengthSource=Input port
      settings: InputPortMap=u0,p1
  cfblk4 : simulink/Discrete/Difference  ICPrevInput=0.0  OutMin=[]  OutMax=[]  OutDataTypeStr=Inherit: Inherit via back propagation  OutDataType=fixdt(1, 16)  OutScaling=2^-10  DoSatur=off
  cfblk5 : DiscreteFilter
  cfblk6 : Delay  ShowEnablePort=on
      settings: InputPortMap=u0,e6
  cfblk7 : If  SampleTime=1
  cyemi_{890..891,897..898,918..928} (15 alike) : DataTypeConversion  OutDataTypeStr=double
  cfblk2 : Outport
  cfblk8 : Outport  Port=2
  cfblk9 : Outport  Port=3
  wires:
  cfblk3/1 -> cfblk8/1, cyemi_890/1
  cfblk10/1(cfblk2) -> cfblk2/1, cyemi_897/1
  cfblk5/1 -> cfblk9/1, cyemi_921/1
  cfblk11/1(cfblk2) -> cyemi_919/1, cyemi_920/1, cyemi_925/1
  cfblk4/1 -> cyemi_918/1, cyemi_922/1, cyemi_928/1
  cfblk7/1 -> cfblk10/Action
  cfblk7/2 -> cfblk11/Action
  cyemi_890/1 -> cfblk10/1(cfblk1)
  cyemi_891/1 -> cfblk10/2(cfblk7)
  cfblk13/1 -> cyemi_891/1
  cyemi_897/1 -> cfblk11/1(cfblk1)
  cyemi_898/1 -> cfblk11/2(cfblk17)
  cfblk15/1 -> cyemi_898/1
  cyemi_918/1 -> cfblk12/1
  cyemi_919/1 -> cfblk13/1
  cyemi_920/1 -> cfblk14/1
  cyemi_921/1 -> cfblk15/1
  cyemi_922/1 -> cfblk3/1
  cyemi_923/1 -> cfblk3/2
  cfblk14/1 -> cyemi_923/1
  cyemi_924/1 -> cfblk4/1
  cfblk6/1 -> cyemi_924/1
  cyemi_925/1 -> cfblk5/1
  cyemi_926/1 -> cfblk6/1
  cfblk12/1 -> cyemi_926/1
  cyemi_927/1 -> cfblk6/2
  cfblk1/1 -> cyemi_927/1
  cyemi_928/1 -> cfblk7/1

== system equivalent/cfblk315 ==
  cfblk1 : Inport
  cfblk8 : Inport  Port=2
  cfblk9 : Inport  Port=3
  cfblk10 : Inport  Port=4
  Action Port : ActionPort  ActionType=then
  cfblk14 : Subsystem  TreatAsAtomicUnit=on
  cfblk15 : Subsystem  TreatAsAtomicUnit=on
  cfblk3 : simulink/Discrete/Transfer Fcn Real Zero  ZeroZ=0.75  ICPrevInput=0.0  DoSatur=off
      settings: SourceProductName=Simulink  SourceProductBaseCode=SL
  cfblk4 : simulink/Discrete/Difference  ICPrevInput=0.0  OutMin=[]  OutMax=[]  OutDataTypeStr=Inherit: Inherit via back propagation  OutDataType=fixdt(1, 16)  OutScaling=2^-10  DoSatur=off
  cfblk5 : UnitDelay  SampleTime=-1
  cfblk6 : DiscreteTransferFcn
  cfblk7 : If  SampleTime=1
  cyemi_{933..934,942..944,950..954} (10 alike) : DataTypeConversion  OutDataTypeStr=double
  cfblk2 : Outport
  cfblk11 : Outport  Port=2
  cfblk12 : Outport  Port=3
  cfblk13 : Outport  Port=4
  wires:
  cfblk9/1 -> cyemi_933/1, cyemi_944/1, cyemi_953/1
  cfblk10/1 -> cyemi_951/1, cyemi_952/1
  cfblk1/1 -> cfblk2/1
  cfblk5/1 -> cfblk13/1
  cfblk15/1(cfblk2) -> cfblk11/1
  cfblk15/2(cfblk10) -> cfblk12/1
  cfblk7/1 -> cfblk14/Action
  cfblk7/2 -> cfblk15/Action
  cyemi_933/1 -> cfblk14/1(cfblk1)
  cyemi_934/1 -> cfblk14/2(cfblk7)
  cfblk6/1 -> cyemi_934/1
  cyemi_942/1 -> cfblk15/1(cfblk1)
  cfblk14/1(cfblk2) -> cyemi_942/1
  cyemi_943/1 -> cfblk15/2(cfblk8)
  cfblk3/1 -> cyemi_943/1
  cyemi_944/1 -> cfblk15/3(cfblk9)
  cyemi_950/1 -> cfblk3/1
  cfblk8/1 -> cyemi_950/1
  cyemi_951/1 -> cfblk4/1
  cyemi_952/1 -> cfblk5/1
  cyemi_953/1 -> cfblk6/1
  cyemi_954/1 -> cfblk7/1
  cfblk4/1 -> cyemi_954/1

== system equivalent/cfblk316 ==
  cfblk1 : Inport
  cfblk9 : Inport  Port=2
  Action Port : ActionPort  ActionType=else
  cfblk3 : simulink/Continuous/PID Controller  Controller=PID  TimeDomain=Discrete-time  SampleTime=-1  IntegratorMethod=Forward Euler  FilterMethod=Forward Euler  Form=Parallel  UseFilter=on  ControllerParametersSource=internal  P=1  I=1  D=0  N=100  InitialConditionSource=internal  InitialConditionForIntegrator=0  InitialConditionForFilter=0  ExternalReset=none  LimitOutput=off  UpperSaturationLimit=inf  LowerSaturationLimit=-inf  LinearizeAsGain=off  AntiWindupMode=none  Kb=1  TrackingMode=off  Kt=1  PParamMin=[]  PParamMax=[]  IParamMin=[]  IParamMax=[]  DParamMin=[]  DParamMax=[]  NParamMin=[]  NParamMax=[]  KbParamMin=[]  KbParamMax=[]  KtParamMin=[]  KtParamMax=[]  POutMin=[]  POutMax=[]  IOutMin=[]  IOutMax=[]  DOutMin=[]  DOutMax=[]  NOutMin=[]  NOutMax=[]  KbOutMin=[]  KbOutMax=[]  KtOutMin=[]  KtOutMax=[]  IntegratorOutMin=[]  IntegratorOutMax=[]  FilterOutMin=[]  FilterOutMax=[]  SumOutMin=[]  SumOutMax=[]  SumI1OutMin=[]  SumI1OutMax=[]  SumI2OutMin=[]  SumI2OutMax=[]  SumI3OutMin=[]  SumI3OutMax=[]  SumDOutMin=[]  SumDOutMax=[]  SaturationOutMin=[]  SaturationOutMax=[]  IntegratorContinuousStateAttributes=''  IntegratorStateMustResolveToSignalObject=off  IntegratorRTWStateStorageClass=Auto  FilterContinuousStateAttributes=''  FilterStateMustResolveToSignalObject=off  FilterRTWStateStorageClass=Auto  DifferentiatorICPrevScaledInput=0  DifferentiatorOutMin=[]  DifferentiatorOutMax=[]  FilterDiffOutCoefMin=[]  FilterDiffOutCoefMax=[]  SumDenOutMin=[]  SumDenOutMax=[]  SumNumOutMin=[]  SumNumOutMax=[]  ReciprocalOutMin=[]  ReciprocalOutMax=[]  DivideOutMin=[]  DivideOutMax=[]  TunerSelectOption=Transfer Function Based (PID Tuner App)
  cfblk4 : DiscreteIntegrator  SampleTime=-1  ICPrevOutput=DiscIntNeverNeededParam  ICPrevScaledInput=DiscIntNeverNeededParam
  cfblk5 : DiscreteIntegrator  SampleTime=-1  ICPrevOutput=DiscIntNeverNeededParam  ICPrevScaledInput=DiscIntNeverNeededParam
  cfblk6 : simulink/Discrete/Transfer Fcn Real Zero  ZeroZ=0.75  ICPrevInput=0.0  DoSatur=off
      settings: SourceProductName=Simulink  SourceProductBaseCode=SL
  cfblk7 : Delay
  cfblk8 : DiscreteStateSpace  SampleTime=-1
  cyemi_{957..962} (6 alike) : DataTypeConversion  OutDataTypeStr=double
  cfblk2 : Outport
  cfblk10 : Outport  Port=2
  cfblk11 : Outport  Port=3
  wires:
  cfblk4/1 -> cyemi_957/1, cyemi_959/1
  cfblk6/1 -> cfblk11/1
  cfblk5/1 -> cfblk2/1
  cfblk1/1 -> cfblk10/1
  cyemi_957/1 -> cfblk3/1
  cyemi_958/1 -> cfblk4/1
  cfblk8/1 -> cyemi_958/1
  cyemi_959/1 -> cfblk5/1
  cyemi_960/1 -> cfblk6/1
  cfblk7/1 -> cyemi_960/1
  cyemi_961/1 -> cfblk7/1
  cfblk3/1 -> cyemi_961/1
  cyemi_962/1 -> cfblk8/1
  cfblk9/1 -> cyemi_962/1

== system equivalent/cfblk317 ==
  cfblk1 : Inport
  Action Port : ActionPort  ActionType=then
  cfblk3 : DiscreteFilter
  cfblk4 : DiscreteZeroPole  Poles=[0 0.5]  Gain=1  SampleTime=-1
  cfblk5 : simulink/Continuous/PID Controller (2DOF)  Controller=PID  TimeDomain=Discrete-time  SampleTime=-1  IntegratorMethod=Forward Euler  FilterMethod=Forward Euler  Form=Parallel  UseFilter=on  ControllerParametersSource=internal  P=1  I=1  D=0  N=100  b=1  c=1  InitialConditionSource=internal  InitialConditionForIntegrator=0  InitialConditionForFilter=0  ExternalReset=none  LimitOutput=off  UpperSaturationLimit=inf  LowerSaturationLimit=-inf  LinearizeAsGain=off  AntiWindupMode=none  Kb=1  TrackingMode=off  Kt=1  PParamMin=[]  PParamMax=[]  IParamMin=[]  IParamMax=[]  DParamMin=[]  DParamMax=[]  NParamMin=[]  NParamMax=[]  bParamMin=[]  bParamMax=[]  cParamMin=[]  cParamMax=[]  KbParamMin=[]  KbParamMax=[]  KtParamMin=[]  KtParamMax=[]  POutMin=[]  POutMax=[]  IOutMin=[]  IOutMax=[]  DOutMin=[]  DOutMax=[]  NOutMin=[]  NOutMax=[]  bOutMin=[]  bOutMax=[]  cOutMin=[]  cOutMax=[]  KbOutMin=[]  KbOutMax=[]  KtOutMin=[]  KtOutMax=[]  IntegratorOutMin=[]  IntegratorOutMax=[]  FilterOutMin=[]  FilterOutMax=[]  SumOutMin=[]  SumOutMax=[]  Sum1OutMin=[]  Sum1OutMax=[]  Sum2OutMin=[]  Sum2OutMax=[]  Sum3OutMin=[]  Sum3OutMax=[]  SumI1OutMin=[]  SumI1OutMax=[]  SumI2OutMin=[]  SumI2OutMax=[]  SumI3OutMin=[]  SumI3OutMax=[]  SumDOutMin=[]  SumDOutMax=[]  SaturationOutMin=[]  SaturationOutMax=[]  IntegratorContinuousStateAttributes=''  IntegratorStateMustResolveToSignalObject=off  IntegratorRTWStateStorageClass=Auto  FilterContinuousStateAttributes=''  FilterStateMustResolveToSignalObject=off  FilterRTWStateStorageClass=Auto  DifferentiatorICPrevScaledInput=0  DifferentiatorOutMin=[]  DifferentiatorOutMax=[]  FilterDiffOutCoefMin=[]  FilterDiffOutCoefMax=[]  SumDenOutMin=[]  SumDenOutMax=[]  SumNumOutMin=[]  SumNumOutMax=[]  ReciprocalOutMin=[]  ReciprocalOutMax=[]  DivideOutMin=[]  DivideOutMax=[]  TunerSelectOption=Transfer Function Based (PID Tuner App)
  cfblk6 : simulink/Discrete/Difference  ICPrevInput=0.0  OutMin=[]  OutMax=[]  OutDataTypeStr=Inherit: Inherit via back propagation  OutDataType=fixdt(1, 16)  OutScaling=2^-10  DoSatur=off
  cfblk8 : Delay
  cyemi_{964..969} (6 alike) : DataTypeConversion  OutDataTypeStr=double
  cfblk2 : Outport
  cfblk7 : Outport  Port=2
  wires:
  cfblk1/1 -> cfblk7/1, cyemi_966/1, cyemi_967/1
  cfblk5/1 -> cfblk2/1
  cyemi_964/1 -> cfblk3/1
  cfblk8/1 -> cyemi_964/1
  cyemi_965/1 -> cfblk4/1
  cfblk3/1 -> cyemi_965/1
  cyemi_966/1 -> cfblk5/1
  cyemi_967/1 -> cfblk5/2
  cyemi_968/1 -> cfblk6/1
  cfblk4/1 -> cyemi_968/1
  cyemi_969/1 -> cfblk8/1
  cfblk6/1 -> cyemi_969/1

== system equivalent/cfblk318 ==
  cfblk1 : Inport
  cfblk11 : Inport  Port=2
  Action Port : ActionPort  ActionType=else
  cfblk10 : DiscreteZeroPole  Poles=[0 0.5]  Gain=1  SampleTime=-1
  cfblk12 : Delay
  cfblk13 : Delay
  cfblk14 : DataTypeConversion  OutDataTypeStr=uint32
  cfblk15 : DataTypeConversion  OutDataTypeStr=double
  cfblk16 : DataTypeConversion  OutDataTypeStr=double
  cfblk17 : DataTypeConversion  OutDataTypeStr=double
  cfblk3 : simulink/Continuous/PID Controller  Controller=PID  TimeDomain=Discrete-time  SampleTime=-1  IntegratorMethod=Forward Euler  FilterMethod=Forward Euler  Form=Parallel  UseFilter=on  ControllerParametersSource=internal  P=1  I=1  D=0  N=100  InitialConditionSource=internal  InitialConditionForIntegrator=0  InitialConditionForFilter=0  ExternalReset=none  LimitOutput=off  UpperSaturationLimit=inf  LowerSaturationLimit=-inf  LinearizeAsGain=off  AntiWindupMode=none  Kb=1  TrackingMode=off  Kt=1  PParamMin=[]  PParamMax=[]  IParamMin=[]  IParamMax=[]  DParamMin=[]  DParamMax=[]  NParamMin=[]  NParamMax=[]  KbParamMin=[]  KbParamMax=[]  KtParamMin=[]  KtParamMax=[]  POutMin=[]  POutMax=[]  IOutMin=[]  IOutMax=[]  DOutMin=[]  DOutMax=[]  NOutMin=[]  NOutMax=[]  KbOutMin=[]  KbOutMax=[]  KtOutMin=[]  KtOutMax=[]  IntegratorOutMin=[]  IntegratorOutMax=[]  FilterOutMin=[]  FilterOutMax=[]  SumOutMin=[]  SumOutMax=[]  SumI1OutMin=[]  SumI1OutMax=[]  SumI2OutMin=[]  SumI2OutMax=[]  SumI3OutMin=[]  SumI3OutMax=[]  SumDOutMin=[]  SumDOutMax=[]  SaturationOutMin=[]  SaturationOutMax=[]  IntegratorContinuousStateAttributes=''  IntegratorStateMustResolveToSignalObject=off  IntegratorRTWStateStorageClass=Auto  FilterContinuousStateAttributes=''  FilterStateMustResolveToSignalObject=off  FilterRTWStateStorageClass=Auto  DifferentiatorICPrevScaledInput=0  DifferentiatorOutMin=[]  DifferentiatorOutMax=[]  FilterDiffOutCoefMin=[]  FilterDiffOutCoefMax=[]  SumDenOutMin=[]  SumDenOutMax=[]  SumNumOutMin=[]  SumNumOutMax=[]  ReciprocalOutMin=[]  ReciprocalOutMax=[]  DivideOutMin=[]  DivideOutMax=[]  TunerSelectOption=Transfer Function Based (PID Tuner App)
  cfblk4 : simulink/Discrete/Transfer Fcn First Order  PoleZ=0.95  ICPrevOutput=0.0  DoSatur=off
      settings: SourceProductName=Simulink
  cfblk5 : Delay
  cfblk6 : Delay  DelayLengthSource=Input port
      settings: InputPortMap=u0,p1
  cfblk7 : simulink/Discrete/Transfer Fcn First Order  PoleZ=0.95  ICPrevOutput=0.0  DoSatur=off
      settings: SourceProductName=Simulink
  cfblk8 : DiscreteTransferFcn
  cfblk9 : DiscreteFilter
  cyemi_{972..973,975..977,979..980,982,984..986} (11 alike) : DataTypeConversion  OutDataTypeStr=double
  cyemi_{974,978,981,983} (4 alike) : DataTypeConversion  OutDataTypeStr=uint32
  cfblk2 : Outport
  wires:
  cfblk1/1 -> cfblk2/1
  cfblk14/1 -> cyemi_974/1, cyemi_983/1
  cyemi_972/1 -> cfblk10/1
  cfblk4/1 -> cyemi_972/1
  cyemi_973/1 -> cfblk12/1
  cfblk10/1 -> cyemi_973/1
  cyemi_974/1 -> cfblk13/1
  cyemi_975/1 -> cfblk14/1
  cfblk8/1 -> cyemi_975/1
  cyemi_976/1 -> cfblk15/1
  cfblk16/1 -> cyemi_976/1
  cyemi_977/1 -> cfblk16/1
  cfblk9/1 -> cyemi_977/1
  cyemi_978/1 -> cfblk17/1
  cfblk5/1 -> cyemi_978/1
  cyemi_979/1 -> cfblk3/1
  cfblk12/1 -> cyemi_979/1
  cyemi_980/1 -> cfblk4/1
  cfblk3/1 -> cyemi_980/1
  cyemi_981/1 -> cfblk5/1
  cfblk13/1 -> cyemi_981/1
  cyemi_982/1 -> cfblk6/1
  cfblk7/1 -> cyemi_982/1
  cyemi_983/1 -> cfblk6/2
  cyemi_984/1 -> cfblk7/1
  cfblk11/1 -> cyemi_984/1
  cyemi_985/1 -> cfblk8/1
  cfblk15/1 -> cyemi_985/1
  cyemi_986/1 -> cfblk9/1
  cfblk17/1 -> cyemi_986/1

== system equivalent/cfblk319 ==
  cfblk1 : Inport
  cfblk14 : Inport  Port=2
  Action Port : ActionPort  ActionType=then
  cfblk10 : DiscreteTransferFcn
  cfblk11 : Delay  ShowEnablePort=on
      settings: InputPortMap=u0,e6
  cfblk12 : DiscreteFilter
  cfblk13 : simulink/Discrete/Difference  ICPrevInput=0.0  OutMin=[]  OutMax=[]  OutDataTypeStr=Inherit: Inherit via back propagation  OutDataType=fixdt(1, 16)  OutScaling=2^-10  DoSatur=off
  cfblk3 : DiscreteIntegrator  SampleTime=-1  ICPrevOutput=DiscIntNeverNeededParam  ICPrevScaledInput=DiscIntNeverNeededParam
  cfblk4 : simulink/Continuous/PID Controller (2DOF)  Controller=PID  TimeDomain=Discrete-time  SampleTime=-1  IntegratorMethod=Forward Euler  FilterMethod=Forward Euler  Form=Parallel  UseFilter=on  ControllerParametersSource=internal  P=1  I=1  D=0  N=100  b=1  c=1  InitialConditionSource=internal  InitialConditionForIntegrator=0  InitialConditionForFilter=0  ExternalReset=none  LimitOutput=off  UpperSaturationLimit=inf  LowerSaturationLimit=-inf  LinearizeAsGain=off  AntiWindupMode=none  Kb=1  TrackingMode=off  Kt=1  PParamMin=[]  PParamMax=[]  IParamMin=[]  IParamMax=[]  DParamMin=[]  DParamMax=[]  NParamMin=[]  NParamMax=[]  bParamMin=[]  bParamMax=[]  cParamMin=[]  cParamMax=[]  KbParamMin=[]  KbParamMax=[]  KtParamMin=[]  KtParamMax=[]  POutMin=[]  POutMax=[]  IOutMin=[]  IOutMax=[]  DOutMin=[]  DOutMax=[]  NOutMin=[]  NOutMax=[]  bOutMin=[]  bOutMax=[]  cOutMin=[]  cOutMax=[]  KbOutMin=[]  KbOutMax=[]  KtOutMin=[]  KtOutMax=[]  IntegratorOutMin=[]  IntegratorOutMax=[]  FilterOutMin=[]  FilterOutMax=[]  SumOutMin=[]  SumOutMax=[]  Sum1OutMin=[]  Sum1OutMax=[]  Sum2OutMin=[]  Sum2OutMax=[]  Sum3OutMin=[]  Sum3OutMax=[]  SumI1OutMin=[]  SumI1OutMax=[]  SumI2OutMin=[]  SumI2OutMax=[]  SumI3OutMin=[]  SumI3OutMax=[]  SumDOutMin=[]  SumDOutMax=[]  SaturationOutMin=[]  SaturationOutMax=[]  IntegratorContinuousStateAttributes=''  IntegratorStateMustResolveToSignalObject=off  IntegratorRTWStateStorageClass=Auto  FilterContinuousStateAttributes=''  FilterStateMustResolveToSignalObject=off  FilterRTWStateStorageClass=Auto  DifferentiatorICPrevScaledInput=0  DifferentiatorOutMin=[]  DifferentiatorOutMax=[]  FilterDiffOutCoefMin=[]  FilterDiffOutCoefMax=[]  SumDenOutMin=[]  SumDenOutMax=[]  SumNumOutMin=[]  SumNumOutMax=[]  ReciprocalOutMin=[]  ReciprocalOutMax=[]  DivideOutMin=[]  DivideOutMax=[]  TunerSelectOption=Transfer Function Based (PID Tuner App)
  cfblk5 : simulink/Continuous/PID Controller  Controller=PID  TimeDomain=Discrete-time  SampleTime=-1  IntegratorMethod=Forward Euler  FilterMethod=Forward Euler  Form=Parallel  UseFilter=on  ControllerParametersSource=internal  P=1  I=1  D=0  N=100  InitialConditionSource=internal  InitialConditionForIntegrator=0  InitialConditionForFilter=0  ExternalReset=none  LimitOutput=off  UpperSaturationLimit=inf  LowerSaturationLimit=-inf  LinearizeAsGain=off  AntiWindupMode=none  Kb=1  TrackingMode=off  Kt=1  PParamMin=[]  PParamMax=[]  IParamMin=[]  IParamMax=[]  DParamMin=[]  DParamMax=[]  NParamMin=[]  NParamMax=[]  KbParamMin=[]  KbParamMax=[]  KtParamMin=[]  KtParamMax=[]  POutMin=[]  POutMax=[]  IOutMin=[]  IOutMax=[]  DOutMin=[]  DOutMax=[]  NOutMin=[]  NOutMax=[]  KbOutMin=[]  KbOutMax=[]  KtOutMin=[]  KtOutMax=[]  IntegratorOutMin=[]  IntegratorOutMax=[]  FilterOutMin=[]  FilterOutMax=[]  SumOutMin=[]  SumOutMax=[]  SumI1OutMin=[]  SumI1OutMax=[]  SumI2OutMin=[]  SumI2OutMax=[]  SumI3OutMin=[]  SumI3OutMax=[]  SumDOutMin=[]  SumDOutMax=[]  SaturationOutMin=[]  SaturationOutMax=[]  IntegratorContinuousStateAttributes=''  IntegratorStateMustResolveToSignalObject=off  IntegratorRTWStateStorageClass=Auto  FilterContinuousStateAttributes=''  FilterStateMustResolveToSignalObject=off  FilterRTWStateStorageClass=Auto  DifferentiatorICPrevScaledInput=0  DifferentiatorOutMin=[]  DifferentiatorOutMax=[]  FilterDiffOutCoefMin=[]  FilterDiffOutCoefMax=[]  SumDenOutMin=[]  SumDenOutMax=[]  SumNumOutMin=[]  SumNumOutMax=[]  ReciprocalOutMin=[]  ReciprocalOutMax=[]  DivideOutMin=[]  DivideOutMax=[]  TunerSelectOption=Transfer Function Based (PID Tuner App)
  cfblk6 : simulink/Discrete/Transfer Fcn Real Zero  ZeroZ=0.75  ICPrevInput=0.0  DoSatur=off
      settings: SourceProductName=Simulink  SourceProductBaseCode=SL
  cfblk7 : DiscreteTransferFcn
  cfblk8 : UnitDelay  SampleTime=-1
  cfblk9 : DiscreteFilter
  cyemi_{989..1001} (13 alike) : DataTypeConversion  OutDataTypeStr=double
  cfblk2 : Outport
  wires:
  cfblk13/1 -> cfblk2/1
  cfblk9/1 -> cyemi_991/1, cyemi_995/1
  cyemi_989/1 -> cfblk10/1
  cfblk11/1 -> cyemi_989/1
  cyemi_990/1 -> cfblk11/1
  cfblk8/1 -> cyemi_990/1
  cyemi_991/1 -> cfblk11/2
  cyemi_992/1 -> cfblk12/1
  cfblk14/1 -> cyemi_992/1
  cyemi_993/1 -> cfblk13/1
  cfblk5/1 -> cyemi_993/1
  cyemi_994/1 -> cfblk3/1
  cfblk7/1 -> cyemi_994/1
  cyemi_995/1 -> cfblk4/1
  cyemi_996/1 -> cfblk4/2
  cfblk12/1 -> cyemi_996/1
  cyemi_997/1 -> cfblk5/1
  cfblk10/1 -> cyemi_997/1
  cyemi_998/1 -> cfblk6/1
  cfblk3/1 -> cyemi_998/1
  cyemi_999/1 -> cfblk7/1
  cfblk1/1 -> cyemi_999/1
  cyemi_1000/1 -> cfblk8/1
  cfblk4/1 -> cyemi_1000/1
  cyemi_1001/1 -> cfblk9/1
  cfblk6/1 -> cyemi_1001/1
